simulink model "Two_Level_Inverter_SPS_lca"  (Simulink 7.8)
settings: Solver=FixedStepDiscrete  StartTime=0.0  StopTime=1  FixedStep=Ts_simulation  RelTol=1e-3
PostLoadFcn:
  | Two_Level_Inverter_params;
InitFcn:
  | Two_Level_Inverter_params;
values from neighbouring files (symbols this model uses):
  Li = 100e-3    (= 0.1)    [Two_Level_Inverter_params.m]
  Ts_simulation = 250e-9    (= 2.5e-07)    [Two_Level_Inverter_params.m]
  U01 = 100    [Two_Level_Inverter_params.m]
libraries: powerlib x14
settings Model: Creator=JeromeCoutel  LastModifiedBy=jonathanbouchard
settings DebuggingCC: UnconnectedInputMsg=none  UnconnectedOutputMsg=none  UnconnectedLineMsg=none
settings CodeAppCC: CustomSymbolStrType=$N$R$M_T
settings GRTTargetCC: TargetFunctionLibrary=NOT IN USE  CPPClassGenCompliant=on

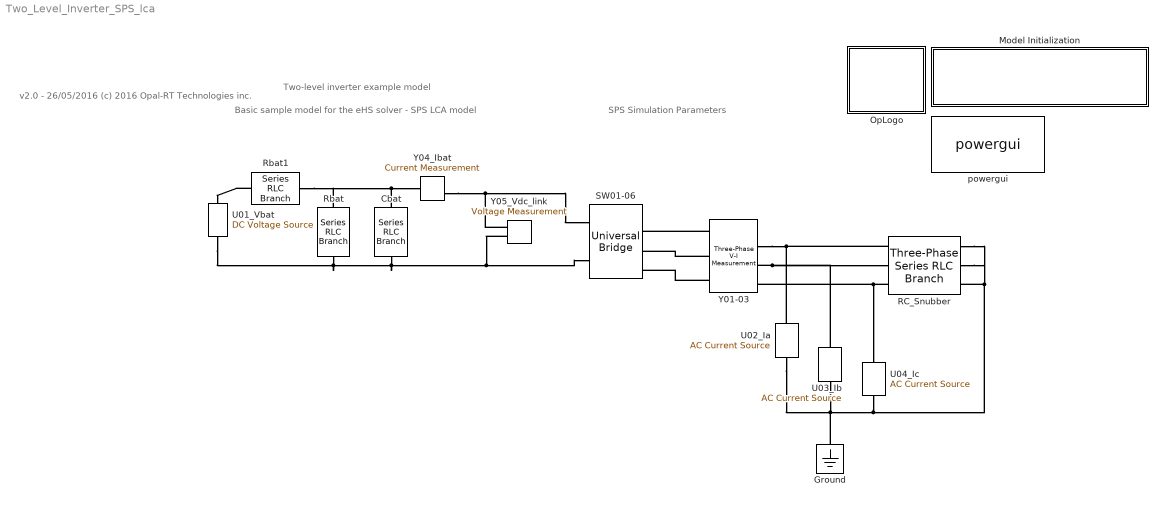
== system Two_Level_Inverter_SPS_lca ==
  note: v2.0 - 26/05/2016
      | (c) 2016 Opal-RT Technologies inc.
  note: Two-level inverter example model
  note: Basic sample model for the eHS solver - SPS LCA model
  note: SPS Simulation Parameters
  Cbat : powerlib/Elements/Series RLC Branch  LConnTagsString=__new0  RConnTagsString=__new0  BranchType=C  Resistance=10000  Inductance=1e-3  SetiL0=off  InitialCurrent=0  Capacitance=0.01  Setx0=off  InitialVoltage=0  Measurements=None
  Ground : powerlib/Elements/Ground  LConnTagsString=a
  Model Initialization : Subsystem
      settings: CopyFcn=set_param(gcb,'LinkStatus','none')
  OpLogo : Subsystem
  RC_Snubber : powerlib/Elements/Three-Phase Series RLC Branch  LConnTagsString=A|B|C  RConnTagsString=A|B|C  BranchType=RC  Resistance=100  Inductance=Li  Capacitance=1e-6  Measurements=None
  Rbat : powerlib/Elements/Series RLC Branch  LConnTagsString=__new0  RConnTagsString=__new0  BranchType=R  Resistance=10000  Inductance=1e-3  SetiL0=off  InitialCurrent=0  Capacitance=1e-6  Setx0=off  InitialVoltage=0  Measurements=None
  Rbat1 : powerlib/Elements/Series RLC Branch  LConnTagsString=__new0  RConnTagsString=__new0  BranchType=R  Resistance=1  Inductance=1e-3  SetiL0=off  InitialCurrent=0  Capacitance=1e-6  Setx0=off  InitialVoltage=0  Measurements=None
  SW01-06 : powerlib/Power Electronics/Universal Bridge  Arms=3  SnubberResistance=Rs  SnubberCapacitance=inf  Device=IGBT / Diodes  Ron=0.01  Lon=0  ForwardVoltages="[  0  0  ]"  ForwardVoltage=0  GTOparameters=[ 10e-6 , 20e-6 ]  IGBTparameters="[  0  0  ]"  Measurements=None  Measurements_2=None  converterType=Rectifier
  U01_Vbat : powerlib/Electrical Sources/DC Voltage Source  Amplitude=U01  Measurements=None
  U02_Ia : powerlib/Electrical Sources/AC Current Source  Amplitude=10  Phase=0  Frequency=60  SampleTime=0  Measurements=None
  U03_Ib : powerlib/Electrical Sources/AC Current Source  Amplitude=10  Phase=0  Frequency=60  SampleTime=0  Measurements=None
  U04_Ic : powerlib/Electrical Sources/AC Current Source  Amplitude=10  Phase=0  Frequency=60  SampleTime=0  Measurements=None
  Y01-03 : powerlib/Measurements/Three-Phase V-I Measurement  VoltageMeasurement=phase-to-ground  SetLabelV=off  LabelV=Vabc  Vpu=off  VpuLL=off  CurrentMeasurement=no  SetLabelI=off  LabelI=Iabc  Ipu=off  Pbase=100e6  Vbase=500e3  OutputType=Complex  PhasorSimulation=off  PSBequivalent=0
  Y04_Ibat : powerlib/Measurements/Current Measurement  PhasorSimulation=off  OutputType=Complex  PSBequivalent=0
  Y05_Vdc_link : powerlib/Measurements/Voltage Measurement  PhasorSimulation=off  OutputType=Complex  PSBequivalent=0
  powergui : powerlib/powergui  Priority=1  SimulationMode=Discrete  SolverType=Tustin  SampleTime=Ts_simulation  frequency=60  SPID=off  DisableSnubberDevices=off  DisableRonSwitches=off  DisableVfSwitches=off  SwTol=0  Interpol=off  DisplayEquations=off  FunctionMessages=off  frequencyindice=0  Pbase=100e6  ErrMax=1e-4  Iterations=50  UnitsV=kV  UnitsW=MW  echomessages=off  HookPort=off  EnableUseOfTLC=off  x0status=blocks  RestoreLinks=warning  ResistiveCurrentMeasurement=off  Frange=[0:2:500]  Ylog=off  Xlog=on  ShowGrid=off  save=off  variable=ZData  structure=ScopeData  ZoomFFT=off  StartTime=7.29  cycles=3  DisplayStyle=1  fundamental=50  FreqAxis=off  MaxFrequency=1000  frequencyindicesteady=1  RmsSteady=1  display=off  Ts=0  methode=off
  connections:
  Y01-03/LConn2 -- SW01-06/LConn2
  Y04_Ibat/RConn1 -- SW01-06/RConn1 -- Y05_Vdc_link/LConn1
  U03_Ib/RConn1 -- Ground/LConn1 -- U04_Ic/RConn1 -- RC_Snubber/RConn1 -- RC_Snubber/RConn2 -- RC_Snubber/RConn3 -- U02_Ia/RConn1
  Y01-03/LConn1 -- SW01-06/LConn1
  Y01-03/LConn3 -- SW01-06/LConn3
  RC_Snubber/LConn1 -- Y01-03/RConn1 -- U02_Ia/LConn1
  Y01-03/RConn2 -- RC_Snubber/LConn2 -- U03_Ib/LConn1
  Cbat/LConn1 -- Rbat1/LConn1 -- Rbat/LConn1 -- Y04_Ibat/LConn1
  Rbat/RConn1 -- U01_Vbat/LConn1 -- Cbat/RConn1 -- SW01-06/RConn2 -- Y05_Vdc_link/LConn2
  Rbat1/RConn1 -- U01_Vbat/RConn1
  RC_Snubber/LConn3 -- U04_Ic/LConn1 -- Y01-03/RConn3

== system Two_Level_Inverter_SPS_lca/Model Initialization ==

== system Two_Level_Inverter_SPS_lca/OpLogo ==
